simulink model "z_relay"  (R2017a)
settings: Solver=VariableStepAuto  StartTime=0.0  StopTime=6  MaxStep=1e-4  RelTol=1e-3
libraries: powerlib x8, powerlib_meascontrol x6, simulink_extras x3, dspstat3 x1
settings Model: Creator=Waqas  LastModifiedBy=ikon

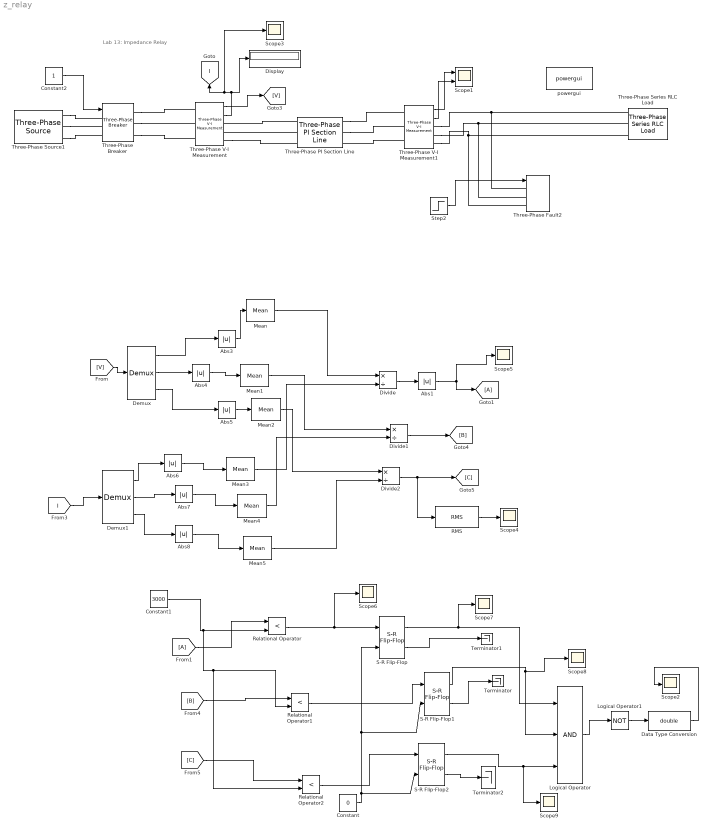
== system z_relay ==
  note: Lab 13:
      | Impedance Relay
  Abs{1,3..8} (7 alike) : Abs
  Constant : Constant  Value=0  OutDataTypeStr=boolean
  Constant1 : Constant  Value=3000
  Constant2 : Constant
  Data Type Conversion : DataTypeConversion  OutDataTypeStr=double
  Demux : Demux  Outputs=3
  Demux1 : Demux  Outputs=3
  Display : Display
  Divide : Product  Inputs=*/
  Divide1 : Product  Inputs=*/
  Divide2 : Product  Inputs=*/
  Logical Operator : Logic  Inputs=3  AllPortsSameDT=off  OutDataTypeStr=boolean
  Logical Operator1 : Logic  Operator=NOT  AllPortsSameDT=off  OutDataTypeStr=boolean
  Mean{,1..5} (6 alike) : powerlib_meascontrol/Measurements/Mean  Freq=60  Vinit=0  Ts=0
  RMS : dspstat3/RMS  run=off  directionMode=Each column  dimension=1  InputProcessing=Columns as channels (frame based)  reset_popup=None
  Relational Operator : RelationalOperator  Operator=<  RndMeth=Simplest
  Relational Operator1 : RelationalOperator  Operator=<  RndMeth=Simplest
  Relational Operator2 : RelationalOperator  Operator=<  RndMeth=Simplest
  S-R Flip-Flop : simulink_extras/Flip Flops/S-R Flip-Flop  initial_condition=0
  S-R Flip-Flop1 : simulink_extras/Flip Flops/S-R Flip-Flop  initial_condition=0
  S-R Flip-Flop2 : simulink_extras/Flip Flops/S-R Flip-Flop  initial_condition=0
  Scope1 : Scope  NumInputPorts=2
  Scope{2..9} (8 alike) : Scope
  Step2 : Step  Time=2  SampleTime=0
  Terminator : Terminator
  Terminator1 : Terminator
  Terminator2 : Terminator
  Three-Phase PI Section Line : powerlib/Elements/Three-Phase PI Section Line  LConnTagsString=a|b|c  RConnTagsString=A|B|C  Frequency=60  Resistances=[ 0.01273 0.3864]  Inductances="[ 0.9337e-3  4.1264e-3]"  Capacitances=[12.74e-9 7.751e-9]  Length=100
      settings: SourceProductName=Simscape Power Systems
  Three-Phase Series RLC Load : powerlib/Elements/Three-Phase Series RLC Load  LConnTagsString=A|B|C  Configuration=Y (grounded)  NominalVoltage=11e3  Vabc=[1e3 1e3 1e3]  Vabcp=[1e3 1e3 1e3]  NominalFrequency=60  UnbalancedPower=off  ActivePower=20000  InductivePower=0  CapacitivePower=0  Pabc=[10e3 9e3 11e3]  QLabc=[100 90 110]  QCabc=[100 90 110]  Pabcp=[10e3 9e3 11e3]  QLabcp=[100 90 110]  QCabcp=[100 90 110]  Measurements=None  LoadType=constant Z
  Three-Phase V-I Measurement : powerlib/Measurements/Three-Phase V-I Measurement  VoltageMeasurement=phase-to-phase  SetLabelV=off  LabelV=Vabc  Vpu=off  VpuLL=off  CurrentMeasurement=yes  SetLabelI=off  LabelI=Iabc  Ipu=off  Pbase=100e6  Vbase=500e3  OutputType=Complex  PhasorSimulation=off  PSBequivalent=0
  Three-Phase V-I Measurement1 : powerlib/Measurements/Three-Phase V-I Measurement  VoltageMeasurement=phase-to-ground  SetLabelV=off  LabelV=Vabc  Vpu=off  VpuLL=off  CurrentMeasurement=yes  SetLabelI=off  LabelI=Iabc  Ipu=off  Pbase=100e6  Vbase=500e3  OutputType=Complex  PhasorSimulation=off  PSBequivalent=0
  Three-Phase Breaker : powerlib/Elements/Three-Phase Breaker  InitialState=closed  SwitchA=on  SwitchB=on  SwitchC=on  SwitchTimes="[1/60  5/60]"  External=on  BreakerResistance=0.01  SnubberResistance=1e6  SnubberCapacitance=inf  Measurements=None
  Three-Phase Fault2 : powerlib/Elements/Three-Phase Fault  InitialStates=0  FaultA=on  FaultB=on  FaultC=on  GroundFault=on  SwitchTimes="[1/60  5/60]"  External=on  SwitchStatus=NaN  FaultResistance=0.001  GroundResistance=0.01  SnubberResistance=1e6  SnubberCapacitance=inf  Measurements=None
  Three-Phase Source1 : powerlib/Electrical Sources/Three-Phase Source  InternalConnection=Yg  VoltagePhases=off  Voltage=11e3  PhaseAngle=0  Voltage_phases=[25e3 25e3 25e3]/sqrt(3)  PhaseAngles_phases=[0 -120 +120]  Frequency=60  NonIdealSource=on  SpecifyImpedance=off  Resistance=0.8929  Inductance=16.58e-3  ShortCircuitLevel=100e6  BaseVoltage=25e3  XRratio=7  BusType=swing  Pref=10e3  Qref=0  Prefabc=[10e3, 10e3, 10e3]  Qrefabc=[0, 0, 0]  Qmin=-inf  Qmax=inf
  powergui : powerlib/powergui  Priority=1  SimulationMode=Continuous  SampleTime=50e-6  frequency=60  Iterations=50  frequencyindice=60  Pbase=100e6  ErrMax=1e-4  UnitsV=kV  UnitsW=MW  buscounter=0  FunctionMessages=off  echomessages=off  EnableUseOfTLC=off  CurrentSourceSwitches=off  DisableSnubberDevices=off  DisableRonSwitches=off  DisableVfSwitches=off  DisplayEquations=off  SolverType=Tustin/Backward Euler (TBE)  Interpol=off  ExternalGateDelay=off  methode=off  Ts=100  x0status=blocks  SPID=on  SwTol=0  HookPort=off  RestoreLinks=warning  ResistiveCurrentMeasurement=off  Frange=[0:2:500]  Ylog=off  Xlog=on  ShowGrid=off  save=off  variable=ZData  structure=0  ZoomFFT=off  StartTime=0.0  cycles=1  DisplayStyle=1  fundamental=60  FreqAxis=off  MaxFrequency=1000  frequencyindicesteady=1  RmsSteady=1  display=off
  tag scope: I=global
  wires:
  Three-Phase V-I Measurement/2 -> [I], Scope3/1, Display/1
  Demux1/2 -> Abs7/1
  Abs4/1 -> Mean1/1
  Abs3/1 -> Mean/1
  [I] -> Demux1/1
  Demux1/3 -> Abs8/1
  [V] -> Demux/1
  Abs5/1 -> Mean2/1
  Demux/2 -> Abs4/1
  Three-Phase V-I Measurement/1 -> [V]
  Three-Phase V-I Measurement1/1 -> Scope1/1
  Three-Phase V-I Measurement1/2 -> Scope1/2
  Step2/1 -> Three-Phase Fault2/1
  Demux/1 -> Abs3/1
  Demux/3 -> Abs5/1
  Demux1/1 -> Abs6/1
  Abs6/1 -> Mean3/1
  Abs7/1 -> Mean4/1
  Abs8/1 -> Mean5/1
  Mean/1 -> Divide/1
  Mean1/1 -> Divide1/1
  Mean2/1 -> Divide2/1
  Mean3/1 -> Divide/2
  Mean4/1 -> Divide1/2
  Mean5/1 -> Divide2/2
  Divide/1 -> Abs1/1
  Divide2/1 -> RMS/1, [C]
  Logical Operator/1 -> Logical Operator1/1
  S-R Flip-Flop/1 -> Scope7/1, Logical Operator/1
  S-R Flip-Flop2/2 -> Terminator2/1
  S-R Flip-Flop1/1 -> Scope8/1, Logical Operator/2
  Data Type Conversion/1 -> Scope2/1
  S-R Flip-Flop1/2 -> Terminator/1
  S-R Flip-Flop2/1 -> Scope9/1, Logical Operator/3
  S-R Flip-Flop/2 -> Terminator1/1
  Relational Operator/1 -> Scope6/1, S-R Flip-Flop/1
  Relational Operator1/1 -> S-R Flip-Flop1/1
  Relational Operator2/1 -> S-R Flip-Flop2/1
  Constant/1 -> S-R Flip-Flop2/2, S-R Flip-Flop1/2, S-R Flip-Flop/2
  [A] -> Relational Operator/1
  [B] -> Relational Operator1/1
  [C] -> Relational Operator2/1
  Constant1/1 -> Relational Operator2/2, Relational Operator1/2, Relational Operator/2
  Divide1/1 -> [B]
  Constant2/1 -> Three-Phase Breaker/1
  RMS/1 -> Scope4/1
  Abs1/1 -> Scope5/1, [A]
  Logical Operator1/1 -> Data Type Conversion/1
  connections:
  Three-Phase Source1/RConn1 -- Three-Phase Breaker/LConn1
  Three-Phase Source1/RConn2 -- Three-Phase Breaker/LConn2
  Three-Phase Source1/RConn3 -- Three-Phase Breaker/LConn3
  Three-Phase Breaker/RConn1 -- Three-Phase V-I Measurement/LConn1
  Three-Phase Breaker/RConn2 -- Three-Phase V-I Measurement/LConn2
  Three-Phase Breaker/RConn3 -- Three-Phase V-I Measurement/LConn3
  Three-Phase PI Section Line/LConn1 -- Three-Phase V-I Measurement/RConn1
  Three-Phase V-I Measurement/RConn3 -- Three-Phase PI Section Line/LConn3
  Three-Phase PI Section Line/RConn1 -- Three-Phase V-I Measurement1/LConn1
  Three-Phase V-I Measurement1/LConn3 -- Three-Phase PI Section Line/RConn3
  Three-Phase V-I Measurement1/RConn1 -- Three-Phase Series RLC Load/LConn1 -- Three-Phase Fault2/LConn1
  Three-Phase V-I Measurement1/RConn2 -- Three-Phase Series RLC Load/LConn2 -- Three-Phase Fault2/LConn2
  Three-Phase V-I Measurement1/RConn3 -- Three-Phase Series RLC Load/LConn3 -- Three-Phase Fault2/LConn3
  Three-Phase PI Section Line/RConn2 -- Three-Phase V-I Measurement1/LConn2
  Three-Phase PI Section Line/LConn2 -- Three-Phase V-I Measurement/RConn2
